simulink model "SF015A_WhlImbRejctn"  (R2013b)
settings: Solver=FixedStepDiscrete  SolverMode=SingleTasking  StartTime=0.0  StopTime=1  FixedStep=0.002  RelTol=1e-3
values from neighbouring files (symbols this model uses):
  ACTIVBANDMAX_ULS_U32 = DataDict.Constant    [SF015A_WhlImbRejctn_DataDict.m]
  ADAPVFILMAX_ULS_F32 = DataDict.Constant    [SF015A_WhlImbRejctn_DataDict.m]
  ARCHGLBPRM_180OVERPI_ULS_F32 = DataDict.Constant    [SF015A_WhlImbRejctn_DataDict.m]
  ARCHGLBPRM_2MILLISEC_SEC_F32 = DataDict.Constant    [SF015A_WhlImbRejctn_DataDict.m]
  ARCHGLBPRM_2PI_ULS_F32 = DataDict.Constant    [SF015A_WhlImbRejctn_DataDict.m]
  ARCHGLBPRM_FLOATZEROTHD_ULS_F32 = DataDict.Constant    [SF015A_WhlImbRejctn_DataDict.m]
  ARCHGLBPRM_PI_ULS_F32 = DataDict.Constant    [SF015A_WhlImbRejctn_DataDict.m]
  ARCHGLBPRM_PIOVER180_ULS_F32 = DataDict.Constant    [SF015A_WhlImbRejctn_DataDict.m]
  ARCHGLBPRM_PIOVER2_ULS_F32 = DataDict.Constant    [SF015A_WhlImbRejctn_DataDict.m]
  CALMINSPERCOUNT_ULS_F32 = DataDict.Constant    [SF015A_WhlImbRejctn_DataDict.m]
  DURATIONDISABLE_CNT_U16 = DataDict.Constant    [SF015A_WhlImbRejctn_DataDict.m]
  FILTWHLSPDMAX_MOTRADPERSEC_F32 = DataDict.Constant    [SF015A_WhlImbRejctn_DataDict.m]
  MICROSECTOMILLISEC_ULS_F32 = DataDict.Constant    [SF015A_WhlImbRejctn_DataDict.m]
  MINSTOMILLISEC_ULS_F32 = DataDict.Constant    [SF015A_WhlImbRejctn_DataDict.m]
  NINETY_ULS_F32 = DataDict.Constant    [SF015A_WhlImbRejctn_DataDict.m]
  NODEBSTEP_CNT_U16 = DataDict.Constant    [SF015A_WhlImbRejctn_DataDict.m]
  NROFDLY_CNT_U08 = DataDict.Constant    [SF015A_WhlImbRejctn_DataDict.m]
  ONEHALF_ULS_F32 = DataDict.Constant    [SF015A_WhlImbRejctn_DataDict.m]
  ONEHUNDRED_ULS_F32 = DataDict.Constant    [SF015A_WhlImbRejctn_DataDict.m]
  ONEOVRTHREE_ULS_F32 = DataDict.Constant    [SF015A_WhlImbRejctn_DataDict.m]
  ONEOVRTWENTY_ULS_F32 = DataDict.Constant    [SF015A_WhlImbRejctn_DataDict.m]
  ONETHOUSAND_ULS_F32 = DataDict.Constant    [SF015A_WhlImbRejctn_DataDict.m]
  PEAKMAX_ULS_F32 = DataDict.Constant    [SF015A_WhlImbRejctn_DataDict.m]
  PEAKMIN_ULS_F32 = DataDict.Constant    [SF015A_WhlImbRejctn_DataDict.m]
  PHAADJMAX_ULS_F32 = DataDict.Constant    [SF015A_WhlImbRejctn_DataDict.m]
  PITIMESSAMPLETIME_ULS_F32 = DataDict.Constant    [SF015A_WhlImbRejctn_DataDict.m]
  STOREDMINSPERCOUNT_ULS_F32 = DataDict.Constant    [SF015A_WhlImbRejctn_DataDict.m]
  TWO_ULS_F32 = DataDict.Constant    [SF015A_WhlImbRejctn_DataDict.m]
  TWOOVRTHREE_ULS_F32 = DataDict.Constant    [SF015A_WhlImbRejctn_DataDict.m]
  WhlImbRejctnAdpvFac = DataDict.Calibration    [SF015A_WhlImbRejctn_DataDict.m]
  WhlImbRejctnAutScaEna = DataDict.Calibration    [SF015A_WhlImbRejctn_DataDict.m]
  WhlImbRejctnAutScaTar = DataDict.Calibration    [SF015A_WhlImbRejctn_DataDict.m]
  WhlImbRejctnCurrMgnSlewPerLoop = DataDict.Calibration    [SF015A_WhlImbRejctn_DataDict.m]
  WhlImbRejctnDcTrendFltRcvryDly = DataDict.Calibration    [SF015A_WhlImbRejctn_DataDict.m]
  WhlImbRejctnDcTrendFltRcvryNegStep = DataDict.Calibration    [SF015A_WhlImbRejctn_DataDict.m]
  WhlImbRejctnDcTrendFltRcvryPosStep = DataDict.Calibration    [SF015A_WhlImbRejctn_DataDict.m]
  WhlImbRejctnDcTrendFltRcvryThd = DataDict.Calibration    [SF015A_WhlImbRejctn_DataDict.m]
  WhlImbRejctnDcTrendTh2Tq = DataDict.Calibration    [SF015A_WhlImbRejctn_DataDict.m]
  WhlImbRejctnDcTrendThTq = DataDict.Calibration    [SF015A_WhlImbRejctn_DataDict.m]
  WhlImbRejctnDcTrendTi2Sec = DataDict.Calibration    [SF015A_WhlImbRejctn_DataDict.m]
  WhlImbRejctnDcTrendTiSec = DataDict.Calibration    [SF015A_WhlImbRejctn_DataDict.m]
  WhlImbRejctnEnaSlewPerLoop = DataDict.Calibration    [SF015A_WhlImbRejctn_DataDict.m]
  WhlImbRejctnFctEna = DataDict.Calibration    [SF015A_WhlImbRejctn_DataDict.m]
  WhlImbRejctnFrqDiagcAmpThd = DataDict.Calibration    [SF015A_WhlImbRejctn_DataDict.m]
  WhlImbRejctnFrqDiagcEna = DataDict.Calibration    [SF015A_WhlImbRejctn_DataDict.m]
  WhlImbRejctnFrqDiagcFltRcvryDly = DataDict.Calibration    [SF015A_WhlImbRejctn_DataDict.m]
  WhlImbRejctnFrqDiagcFltRcvryNegStep = DataDict.Calibration    [SF015A_WhlImbRejctn_DataDict.m]
  WhlImbRejctnFrqDiagcFltRcvryPosStep = DataDict.Calibration    [SF015A_WhlImbRejctn_DataDict.m]
  WhlImbRejctnFrqDiagcFltRcvryThd = DataDict.Calibration    [SF015A_WhlImbRejctn_DataDict.m]
  WhlImbRejctnFrqDiagcThd = DataDict.Calibration    [SF015A_WhlImbRejctn_DataDict.m]
  WhlImbRejctnFrqDiagcTout = DataDict.Calibration    [SF015A_WhlImbRejctn_DataDict.m]
  WhlImbRejctnFrqDiagcUgrPoleMgn = DataDict.Calibration    [SF015A_WhlImbRejctn_DataDict.m]
  WhlImbRejctnFrqScaTblX = DataDict.Calibration    [SF015A_WhlImbRejctn_DataDict.m]
  WhlImbRejctnMaxDurn = DataDict.Calibration    [SF015A_WhlImbRejctn_DataDict.m]
  WhlImbRejctnMaxMgn = DataDict.Calibration    [SF015A_WhlImbRejctn_DataDict.m]
  WhlImbRejctnMaxMgnFltNegStep = DataDict.Calibration    [SF015A_WhlImbRejctn_DataDict.m]
  WhlImbRejctnMaxMgnFltPosStep = DataDict.Calibration    [SF015A_WhlImbRejctn_DataDict.m]
  WhlImbRejctnMaxMgnFltRcvryDly = DataDict.Calibration    [SF015A_WhlImbRejctn_DataDict.m]
  WhlImbRejctnMaxMgnFltRcvryNegStep = DataDict.Calibration    [SF015A_WhlImbRejctn_DataDict.m]
  WhlImbRejctnMaxMgnFltRcvryPosStep = DataDict.Calibration    [SF015A_WhlImbRejctn_DataDict.m]
  WhlImbRejctnMaxMgnFltRcvryThd = DataDict.Calibration    [SF015A_WhlImbRejctn_DataDict.m]
  WhlImbRejctnMaxMgnFltThd = DataDict.Calibration    [SF015A_WhlImbRejctn_DataDict.m]
  WhlImbRejctnMgnEstimnDeltaSca = DataDict.Calibration    [SF015A_WhlImbRejctn_DataDict.m]
  WhlImbRejctnMgnEstimnDiThd = DataDict.Calibration    [SF015A_WhlImbRejctn_DataDict.m]
  WhlImbRejctnMgnEstimnEnaThd = DataDict.Calibration    [SF015A_WhlImbRejctn_DataDict.m]
  WhlImbRejctnMgnEstimnFrq = DataDict.Calibration    [SF015A_WhlImbRejctn_DataDict.m]
  WhlImbRejctnMgnEstimnFrqDelta = DataDict.Calibration    [SF015A_WhlImbRejctn_DataDict.m]
  WhlImbRejctnMgnEstimnLeak = DataDict.Calibration    [SF015A_WhlImbRejctn_DataDict.m]
  WhlImbRejctnRampDwnTi = DataDict.Calibration    [SF015A_WhlImbRejctn_DataDict.m]
  WhlImbRejctnScaCncl = DataDict.Calibration    [SF015A_WhlImbRejctn_DataDict.m]
  WhlImbRejctnUgrPoleMgn = DataDict.Calibration    [SF015A_WhlImbRejctn_DataDict.m]
  WhlImbRejctnVehSpdEna = DataDict.Calibration    [SF015A_WhlImbRejctn_DataDict.m]
  WhlImbRejctnWhlSpdCorrlnFltRcvryDly = DataDict.Calibration    [SF015A_WhlImbRejctn_DataDict.m]
  WhlImbRejctnWhlSpdCorrlnFltRcvryNegStep = DataDict.Calibration    [SF015A_WhlImbRejctn_DataDict.m]
  WhlImbRejctnWhlSpdCorrlnFltRcvryPosStep = DataDict.Calibration    [SF015A_WhlImbRejctn_DataDict.m]
  WhlImbRejctnWhlSpdCorrlnFltRcvryThd = DataDict.Calibration    [SF015A_WhlImbRejctn_DataDict.m]
  WhlImbRejctnWhlSpdCorrlnThd = DataDict.Calibration    [SF015A_WhlImbRejctn_DataDict.m]
  WhlImbRejctnWhlSpdCorrlnTi = DataDict.Calibration    [SF015A_WhlImbRejctn_DataDict.m]
  WIRCMDMAX_MOTNWTMTR_F32 = DataDict.Constant    [SF015A_WhlImbRejctn_DataDict.m]
  ZERO_ULS_F32 = DataDict.Constant    [SF015A_WhlImbRejctn_DataDict.m]
undefined symbols (not defined in the file or in its folder): Cntr, NtcNr1, NvmGetErrSts1, SigQlfr1, Sts, SysSt1
libraries: simulink x32, FixdToFloat x32, Fil x20, NxtrLim x15, NxtrNvM x12, NxtrAbslt x8, NxtrMath x7, NxtrMax x6, NxtrMin x4, FloatToFixd x2, LnrIntrpn x2, NxtrSign x1
(part 2 of 12)

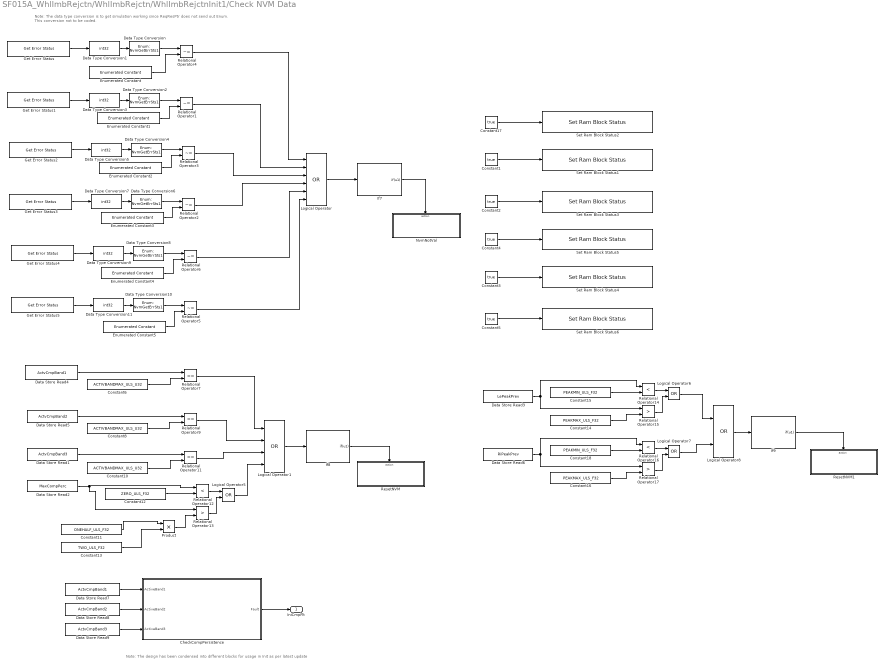
== system SF015A_WhlImbRejctn/WhlImbRejctn/WhlImbRejctnInit1/Check NVM Data ==
  note: Note: The data type conversion is to get simulation working since ReqResPtr does not send out Enum. This
      | conversion not to be coded.
  note: Note: The design has been condensed into different blocks for usage in Init as per latest update
  CheckCompPersistence : Subsystem
  Constant{1..5,17} (6 alike) : Constant  Value=true  OutDataTypeStr=boolean
      settings: AttributesFormatString=%<OutDataTypeStr>
  Constant10 : Constant  RequirementInfo="{'linktype_rmi_doors' '0000ba59 (/E-STEER Core/SubSystem Specifications/Application Functions/SF011A Learned EOT Limits)' '#SF011A_70' 'true' 'REQ:  SF011A_70' '' ; 'linktype_rmi_doors' '0000ba59 (/E-STEER Core/SubSystem Specifications/Application Functions/SF011A Learned EOT Limits)' '#SF011A_71' 'true' 'REQ:  SF011A_71' '' ; 'linktype_rmi_doors' '0000ba59 (/E-STEER Core/SubSystem Specifications/Application Functions/SF011A Learned EOT Limits)' '#SF011A_49' 'true' 'REQ:  SF011A_49' '' } %GIDa_dac22d33_84e0_4d43_9baa_6580695156ec"  Value=ACTIVBANDMAX_ULS_U32
  Constant11 : Constant  RequirementInfo="{'linktype_rmi_doors' '0000ba59 (/E-STEER Core/SubSystem Specifications/Application Functions/SF011A Learned EOT Limits)' '#SF011A_70' 'true' 'REQ:  SF011A_70' '' ; 'linktype_rmi_doors' '0000ba59 (/E-STEER Core/SubSystem Specifications/Application Functions/SF011A Learned EOT Limits)' '#SF011A_71' 'true' 'REQ:  SF011A_71' '' ; 'linktype_rmi_doors' '0000ba59 (/E-STEER Core/SubSystem Specifications/Application Functions/SF011A Learned EOT Limits)' '#SF011A_49' 'true' 'REQ:  SF011A_49' '' } %GIDa_b70b5de3_e4e7_4656_8a10_81d881ba1c41"  Value=ONEHALF_ULS_F32
  Constant12 : Constant  RequirementInfo="{'linktype_rmi_doors' '0000ba59 (/E-STEER Core/SubSystem Specifications/Application Functions/SF011A Learned EOT Limits)' '#SF011A_70' 'true' 'REQ:  SF011A_70' '' ; 'linktype_rmi_doors' '0000ba59 (/E-STEER Core/SubSystem Specifications/Application Functions/SF011A Learned EOT Limits)' '#SF011A_71' 'true' 'REQ:  SF011A_71' '' ; 'linktype_rmi_doors' '0000ba59 (/E-STEER Core/SubSystem Specifications/Application Functions/SF011A Learned EOT Limits)' '#SF011A_48' 'true' 'REQ:  SF011A_48' '' } %GIDa_d9980660_ddd4_4231_a48f_0f3c433b1d8f"  Value=ZERO_ULS_F32
  Constant13 : Constant  RequirementInfo="{'linktype_rmi_doors' '0000ba59 (/E-STEER Core/SubSystem Specifications/Application Functions/SF011A Learned EOT Limits)' '#SF011A_70' 'true' 'REQ:  SF011A_70' '' ; 'linktype_rmi_doors' '0000ba59 (/E-STEER Core/SubSystem Specifications/Application Functions/SF011A Learned EOT Limits)' '#SF011A_71' 'true' 'REQ:  SF011A_71' '' ; 'linktype_rmi_doors' '0000ba59 (/E-STEER Core/SubSystem Specifications/Application Functions/SF011A Learned EOT Limits)' '#SF011A_49' 'true' 'REQ:  SF011A_49' '' } %GIDa_8a202516_8579_4314_b780_b551ef6a9ea7"  Value=TWO_ULS_F32
  Constant14 : Constant  RequirementInfo="{'linktype_rmi_doors' '0000ba59 (/E-STEER Core/SubSystem Specifications/Application Functions/SF011A Learned EOT Limits)' '#SF011A_70' 'true' 'REQ:  SF011A_70' '' ; 'linktype_rmi_doors' '0000ba59 (/E-STEER Core/SubSystem Specifications/Application Functions/SF011A Learned EOT Limits)' '#SF011A_71' 'true' 'REQ:  SF011A_71' '' ; 'linktype_rmi_doors' '0000ba59 (/E-STEER Core/SubSystem Specifications/Application Functions/SF011A Learned EOT Limits)' '#SF011A_49' 'true' 'REQ:  SF011A_49' '' } %GIDa_73aa9993_742b_457a_81a0_f953eb76670e"  Value=PEAKMAX_ULS_F32
  Constant15 : Constant  RequirementInfo="{'linktype_rmi_doors' '0000ba59 (/E-STEER Core/SubSystem Specifications/Application Functions/SF011A Learned EOT Limits)' '#SF011A_70' 'true' 'REQ:  SF011A_70' '' ; 'linktype_rmi_doors' '0000ba59 (/E-STEER Core/SubSystem Specifications/Application Functions/SF011A Learned EOT Limits)' '#SF011A_71' 'true' 'REQ:  SF011A_71' '' ; 'linktype_rmi_doors' '0000ba59 (/E-STEER Core/SubSystem Specifications/Application Functions/SF011A Learned EOT Limits)' '#SF011A_48' 'true' 'REQ:  SF011A_48' '' } %GIDa_1412b3b4_8a5a_4483_b46c_39b8aea63137"  Value=PEAKMIN_ULS_F32
  Constant16 : Constant  RequirementInfo="{'linktype_rmi_doors' '0000ba59 (/E-STEER Core/SubSystem Specifications/Application Functions/SF011A Learned EOT Limits)' '#SF011A_70' 'true' 'REQ:  SF011A_70' '' ; 'linktype_rmi_doors' '0000ba59 (/E-STEER Core/SubSystem Specifications/Application Functions/SF011A Learned EOT Limits)' '#SF011A_71' 'true' 'REQ:  SF011A_71' '' ; 'linktype_rmi_doors' '0000ba59 (/E-STEER Core/SubSystem Specifications/Application Functions/SF011A Learned EOT Limits)' '#SF011A_49' 'true' 'REQ:  SF011A_49' '' } %GIDa_fb2105b3_9180_4cca_ab02_2c62039e61f3"  Value=PEAKMAX_ULS_F32
  Constant18 : Constant  RequirementInfo="{'linktype_rmi_doors' '0000ba59 (/E-STEER Core/SubSystem Specifications/Application Functions/SF011A Learned EOT Limits)' '#SF011A_70' 'true' 'REQ:  SF011A_70' '' ; 'linktype_rmi_doors' '0000ba59 (/E-STEER Core/SubSystem Specifications/Application Functions/SF011A Learned EOT Limits)' '#SF011A_71' 'true' 'REQ:  SF011A_71' '' ; 'linktype_rmi_doors' '0000ba59 (/E-STEER Core/SubSystem Specifications/Application Functions/SF011A Learned EOT Limits)' '#SF011A_48' 'true' 'REQ:  SF011A_48' '' } %GIDa_e66c83e2_3c4a_4c53_aaa1_18a5c79d3e74"  Value=PEAKMIN_ULS_F32
  Constant6 : Constant  RequirementInfo="{'linktype_rmi_doors' '0000ba59 (/E-STEER Core/SubSystem Specifications/Application Functions/SF011A Learned EOT Limits)' '#SF011A_70' 'true' 'REQ:  SF011A_70' '' ; 'linktype_rmi_doors' '0000ba59 (/E-STEER Core/SubSystem Specifications/Application Functions/SF011A Learned EOT Limits)' '#SF011A_71' 'true' 'REQ:  SF011A_71' '' ; 'linktype_rmi_doors' '0000ba59 (/E-STEER Core/SubSystem Specifications/Application Functions/SF011A Learned EOT Limits)' '#SF011A_49' 'true' 'REQ:  SF011A_49' '' } %GIDa_8360f5ba_58c9_48ae_bbc1_d6eb240405df"  Value=ACTIVBANDMAX_ULS_U32
  Constant8 : Constant  RequirementInfo="{'linktype_rmi_doors' '0000ba59 (/E-STEER Core/SubSystem Specifications/Application Functions/SF011A Learned EOT Limits)' '#SF011A_70' 'true' 'REQ:  SF011A_70' '' ; 'linktype_rmi_doors' '0000ba59 (/E-STEER Core/SubSystem Specifications/Application Functions/SF011A Learned EOT Limits)' '#SF011A_71' 'true' 'REQ:  SF011A_71' '' ; 'linktype_rmi_doors' '0000ba59 (/E-STEER Core/SubSystem Specifications/Application Functions/SF011A Learned EOT Limits)' '#SF011A_49' 'true' 'REQ:  SF011A_49' '' } %GIDa_5c7deeb0_1ebc_45b4_93cb_ec8df33bc324"  Value=ACTIVBANDMAX_ULS_U32
  Data Store Read1 : DataStoreRead  RequirementInfo="{'linktype_rmi_doors' '0000ba59 (/E-STEER Core/SubSystem Specifications/Application Functions/SF011A Learned EOT Limits)' '#SF011A_70' 'true' 'REQ:  SF011A_70' '' ; 'linktype_rmi_doors' '0000ba59 (/E-STEER Core/SubSystem Specifications/Application Functions/SF011A Learned EOT Limits)' '#SF011A_71' 'true' 'REQ:  SF011A_71' '' } %GIDa_ec34064d_8d90_476a_a13b_dfcebb6e1578"  DataStoreName=ActvCmpBand3
  Data Store Read2 : DataStoreRead  RequirementInfo="{'linktype_rmi_doors' '0000ba59 (/E-STEER Core/SubSystem Specifications/Application Functions/SF011A Learned EOT Limits)' '#SF011A_70' 'true' 'REQ:  SF011A_70' '' ; 'linktype_rmi_doors' '0000ba59 (/E-STEER Core/SubSystem Specifications/Application Functions/SF011A Learned EOT Limits)' '#SF011A_71' 'true' 'REQ:  SF011A_71' '' } %GIDa_c9bc2b23_4b2d_4415_bc50_be739cb942b2"  DataStoreName=MaxCompPerc
  Data Store Read3 : DataStoreRead  RequirementInfo="{'linktype_rmi_doors' '0000ba59 (/E-STEER Core/SubSystem Specifications/Application Functions/SF011A Learned EOT Limits)' '#SF011A_70' 'true' 'REQ:  SF011A_70' '' ; 'linktype_rmi_doors' '0000ba59 (/E-STEER Core/SubSystem Specifications/Application Functions/SF011A Learned EOT Limits)' '#SF011A_71' 'true' 'REQ:  SF011A_71' '' } %GIDa_b09638af_4375_4cc5_b3f9_eff43fa8b240"  DataStoreName=LePeakPrev
  Data Store Read4 : DataStoreRead  RequirementInfo="{'linktype_rmi_doors' '0000ba59 (/E-STEER Core/SubSystem Specifications/Application Functions/SF011A Learned EOT Limits)' '#SF011A_70' 'true' 'REQ:  SF011A_70' '' ; 'linktype_rmi_doors' '0000ba59 (/E-STEER Core/SubSystem Specifications/Application Functions/SF011A Learned EOT Limits)' '#SF011A_71' 'true' 'REQ:  SF011A_71' '' } %GIDa_a896886f_cd25_4b88_9045_5429e28523e8"  DataStoreName=ActvCmpBand1
  Data Store Read5 : DataStoreRead  RequirementInfo="{'linktype_rmi_doors' '0000ba59 (/E-STEER Core/SubSystem Specifications/Application Functions/SF011A Learned EOT Limits)' '#SF011A_70' 'true' 'REQ:  SF011A_70' '' ; 'linktype_rmi_doors' '0000ba59 (/E-STEER Core/SubSystem Specifications/Application Functions/SF011A Learned EOT Limits)' '#SF011A_71' 'true' 'REQ:  SF011A_71' '' } %GIDa_49f944b4_3c4a_4d70_b0f8_71dc9df1d416"  DataStoreName=ActvCmpBand2
  Data Store Read6 : DataStoreRead  RequirementInfo="{'linktype_rmi_doors' '0000ba59 (/E-STEER Core/SubSystem Specifications/Application Functions/SF011A Learned EOT Limits)' '#SF011A_70' 'true' 'REQ:  SF011A_70' '' ; 'linktype_rmi_doors' '0000ba59 (/E-STEER Core/SubSystem Specifications/Application Functions/SF011A Learned EOT Limits)' '#SF011A_71' 'true' 'REQ:  SF011A_71' '' } %GIDa_db267250_3306_4bc6_b10d_eb14da1fa863"  DataStoreName=RiPeakPrev
  Data Store Read7 : DataStoreRead  Priority=3  DataStoreName=ActvCmpBand1
      settings: AttributesFormatString=Priority=%<Priority>
  Data Store Read8 : DataStoreRead  Priority=3  DataStoreName=ActvCmpBand2
      settings: AttributesFormatString=Priority=%<Priority>
  Data Store Read9 : DataStoreRead  Priority=3  DataStoreName=ActvCmpBand3
      settings: AttributesFormatString=Priority=%<Priority>
  Data Type Conversion : DataTypeConversion  RequirementInfo="{'linktype_rmi_doors' '0000ba59 (/E-STEER Core/SubSystem Specifications/Application Functions/SF011A Learned EOT Limits)' '#SF011A_124' 'true' 'REQ:  SF011A_124' '' } %GIDa_40af021a_ef54_4ec7_b6de_237be91b60fa"  OutDataTypeStr=Enum: NvmGetErrSts1
  Data Type Conversion1 : DataTypeConversion  RequirementInfo="{'linktype_rmi_doors' '0000ba59 (/E-STEER Core/SubSystem Specifications/Application Functions/SF011A Learned EOT Limits)' '#SF011A_124' 'true' 'REQ:  SF011A_124' '' } %GIDa_97cfbfab_5bcd_4235_a187_9f25ba5a5ff5"  OutDataTypeStr=int32
  Data Type Conversion10 : DataTypeConversion  RequirementInfo="{'linktype_rmi_doors' '0000ba59 (/E-STEER Core/SubSystem Specifications/Application Functions/SF011A Learned EOT Limits)' '#SF011A_124' 'true' 'REQ:  SF011A_124' '' } %GIDa_d1594883_ae26_4fe8_b2c9_9956f34c5b40"  OutDataTypeStr=Enum: NvmGetErrSts1
  Data Type Conversion11 : DataTypeConversion  RequirementInfo="{'linktype_rmi_doors' '0000ba59 (/E-STEER Core/SubSystem Specifications/Application Functions/SF011A Learned EOT Limits)' '#SF011A_124' 'true' 'REQ:  SF011A_124' '' } %GIDa_86b4411a_f525_417b_8f1b_33407c25bf86"  OutDataTypeStr=int32
  Data Type Conversion2 : DataTypeConversion  RequirementInfo="{'linktype_rmi_doors' '0000ba59 (/E-STEER Core/SubSystem Specifications/Application Functions/SF011A Learned EOT Limits)' '#SF011A_124' 'true' 'REQ:  SF011A_124' '' } %GIDa_71155e7c_4e44_40ff_94f4_b9d7723c530e"  OutDataTypeStr=Enum: NvmGetErrSts1
  Data Type Conversion3 : DataTypeConversion  RequirementInfo="{'linktype_rmi_doors' '0000ba59 (/E-STEER Core/SubSystem Specifications/Application Functions/SF011A Learned EOT Limits)' '#SF011A_124' 'true' 'REQ:  SF011A_124' '' } %GIDa_b9c1508a_f5ac_4de0_ab2d_9795f69e770d"  OutDataTypeStr=int32
  Data Type Conversion4 : DataTypeConversion  RequirementInfo="{'linktype_rmi_doors' '0000ba59 (/E-STEER Core/SubSystem Specifications/Application Functions/SF011A Learned EOT Limits)' '#SF011A_124' 'true' 'REQ:  SF011A_124' '' } %GIDa_abad9cc4_b739_49e2_b051_31edac34df3e"  OutDataTypeStr=Enum: NvmGetErrSts1
  Data Type Conversion5 : DataTypeConversion  RequirementInfo="{'linktype_rmi_doors' '0000ba59 (/E-STEER Core/SubSystem Specifications/Application Functions/SF011A Learned EOT Limits)' '#SF011A_124' 'true' 'REQ:  SF011A_124' '' } %GIDa_63d91e5a_8420_42e2_a9f3_80e22cdf1e1c"  OutDataTypeStr=int32
  Data Type Conversion6 : DataTypeConversion  RequirementInfo="{'linktype_rmi_doors' '0000ba59 (/E-STEER Core/SubSystem Specifications/Application Functions/SF011A Learned EOT Limits)' '#SF011A_124' 'true' 'REQ:  SF011A_124' '' } %GIDa_6d191fbc_fa3c_4609_af11_f3505129a929"  OutDataTypeStr=Enum: NvmGetErrSts1
  Data Type Conversion7 : DataTypeConversion  RequirementInfo="{'linktype_rmi_doors' '0000ba59 (/E-STEER Core/SubSystem Specifications/Application Functions/SF011A Learned EOT Limits)' '#SF011A_124' 'true' 'REQ:  SF011A_124' '' } %GIDa_257ee758_1562_45cc_b25c_78b92d5b7d32"  OutDataTypeStr=int32
  Data Type Conversion8 : DataTypeConversion  RequirementInfo="{'linktype_rmi_doors' '0000ba59 (/E-STEER Core/SubSystem Specifications/Application Functions/SF011A Learned EOT Limits)' '#SF011A_124' 'true' 'REQ:  SF011A_124' '' } %GIDa_a7c9a5b3_e719_4c4f_b06f_c23b0932ba59"  OutDataTypeStr=Enum: NvmGetErrSts1
  Data Type Conversion9 : DataTypeConversion  RequirementInfo="{'linktype_rmi_doors' '0000ba59 (/E-STEER Core/SubSystem Specifications/Application Functions/SF011A Learned EOT Limits)' '#SF011A_124' 'true' 'REQ:  SF011A_124' '' } %GIDa_0f1e9d57_eff5_4620_a47c_e9abcc1d02d7"  OutDataTypeStr=int32
  Enumerated Constant : simulink/Sources/Enumerated Constant  RequirementInfo="{'linktype_rmi_doors' '0000ba59 (/E-STEER Core/SubSystem Specifications/Application Functions/SF011A Learned EOT Limits)' '#SF011A_124' 'true' 'REQ:  SF011A_124' '' } %GIDa_d56addf7_f0d4_4bf6_af4c_9a6eaaf5d064"  OutDataTypeStr=Enum: NvmGetErrSts1  Value=NvmGetErrSts1.REQUEST_OK  SampleTime=inf
  Enumerated Constant1 : simulink/Sources/Enumerated Constant  RequirementInfo="{'linktype_rmi_doors' '0000ba59 (/E-STEER Core/SubSystem Specifications/Application Functions/SF011A Learned EOT Limits)' '#SF011A_124' 'true' 'REQ:  SF011A_124' '' } %GIDa_5e154709_209f_4b86_818d_2a89bf246dcb"  OutDataTypeStr=Enum: NvmGetErrSts1  Value=NvmGetErrSts1.REQUEST_OK  SampleTime=inf
  Enumerated Constant2 : simulink/Sources/Enumerated Constant  RequirementInfo="{'linktype_rmi_doors' '0000ba59 (/E-STEER Core/SubSystem Specifications/Application Functions/SF011A Learned EOT Limits)' '#SF011A_124' 'true' 'REQ:  SF011A_124' '' } %GIDa_b9f04514_19b2_47ae_b701_837fe354ebc7"  OutDataTypeStr=Enum: NvmGetErrSts1  Value=NvmGetErrSts1.REQUEST_OK  SampleTime=inf
  Enumerated Constant3 : simulink/Sources/Enumerated Constant  RequirementInfo="{'linktype_rmi_doors' '0000ba59 (/E-STEER Core/SubSystem Specifications/Application Functions/SF011A Learned EOT Limits)' '#SF011A_124' 'true' 'REQ:  SF011A_124' '' } %GIDa_006fb6d4_b105_4186_b45b_bb6a02141efd"  OutDataTypeStr=Enum: NvmGetErrSts1  Value=NvmGetErrSts1.REQUEST_OK  SampleTime=inf
  Enumerated Constant4 : simulink/Sources/Enumerated Constant  RequirementInfo="{'linktype_rmi_doors' '0000ba59 (/E-STEER Core/SubSystem Specifications/Application Functions/SF011A Learned EOT Limits)' '#SF011A_124' 'true' 'REQ:  SF011A_124' '' } %GIDa_f995986c_c311_4ae9_af99_76f05a8496d8"  OutDataTypeStr=Enum: NvmGetErrSts1  Value=NvmGetErrSts1.REQUEST_OK  SampleTime=inf
  Enumerated Constant5 : simulink/Sources/Enumerated Constant  RequirementInfo="{'linktype_rmi_doors' '0000ba59 (/E-STEER Core/SubSystem Specifications/Application Functions/SF011A Learned EOT Limits)' '#SF011A_124' 'true' 'REQ:  SF011A_124' '' } %GIDa_f15c7506_b69b_4bb1_898d_0e3ef15f7387"  OutDataTypeStr=Enum: NvmGetErrSts1  Value=NvmGetErrSts1.REQUEST_OK  SampleTime=inf
  Get Error Status : NxtrNvM/Get Error Status  RequirementInfo="{'linktype_rmi_doors' '0000ba59 (/E-STEER Core/SubSystem Specifications/Application Functions/SF011A Learned EOT Limits)' '#SF011A_124' 'true' 'REQ:  SF011A_124' '' } %GIDa_553b790d_fe60_40ec_8b91_d9fbb8c02471"  FuncName=Get Error Status  NvMBlockName=ActvCmpBand1  VoidFuncRtn=on  ReqResPtr_DSN=NvMGES_ReqResPtr1  Return_DSN=NvMGES_Return
      settings: AttributesFormatString=%<FuncName>
  Get Error Status1 : NxtrNvM/Get Error Status  RequirementInfo="{'linktype_rmi_doors' '0000ba59 (/E-STEER Core/SubSystem Specifications/Application Functions/SF011A Learned EOT Limits)' '#SF011A_124' 'true' 'REQ:  SF011A_124' '' } %GIDa_2abd0d7c_8999_4277_934d_b39154cf423f"  FuncName=Get Error Status  NvMBlockName=ActvCmpBand2  VoidFuncRtn=on  ReqResPtr_DSN=NvMGES_ReqResPtr2  Return_DSN=NvMGES_Return
      settings: AttributesFormatString=%<FuncName>
  Get Error Status2 : NxtrNvM/Get Error Status  RequirementInfo="{'linktype_rmi_doors' '0000ba59 (/E-STEER Core/SubSystem Specifications/Application Functions/SF011A Learned EOT Limits)' '#SF011A_124' 'true' 'REQ:  SF011A_124' '' } %GIDa_b704cbe0_0ff9_45ea_89ac_8ddce2b05c13"  FuncName=Get Error Status  NvMBlockName=ActvCmpBand3  VoidFuncRtn=on  ReqResPtr_DSN=NvMGES_ReqResPtr3  Return_DSN=NvMGES_Return
      settings: AttributesFormatString=%<FuncName>
  Get Error Status3 : NxtrNvM/Get Error Status  RequirementInfo="{'linktype_rmi_doors' '0000ba59 (/E-STEER Core/SubSystem Specifications/Application Functions/SF011A Learned EOT Limits)' '#SF011A_124' 'true' 'REQ:  SF011A_124' '' } %GIDa_06d65f98_25d9_49e6_9db6_cd70c37fa23a"  FuncName=Get Error Status  NvMBlockName=LePeakPrev  VoidFuncRtn=on  ReqResPtr_DSN=NvMGES_ReqResPtr4  Return_DSN=NvMGES_Return
      settings: AttributesFormatString=%<FuncName>
  Get Error Status4 : NxtrNvM/Get Error Status  RequirementInfo="{'linktype_rmi_doors' '0000ba59 (/E-STEER Core/SubSystem Specifications/Application Functions/SF011A Learned EOT Limits)' '#SF011A_124' 'true' 'REQ:  SF011A_124' '' } %GIDa_0df4cd3c_6ba5_402f_93b7_8579f841a241"  FuncName=Get Error Status  NvMBlockName=MaxCompPerc  VoidFuncRtn=on  ReqResPtr_DSN=NvMGES_ReqResPtr5  Return_DSN=NvMGES_Return
      settings: AttributesFormatString=%<FuncName>
  Get Error Status5 : NxtrNvM/Get Error Status  RequirementInfo="{'linktype_rmi_doors' '0000ba59 (/E-STEER Core/SubSystem Specifications/Application Functions/SF011A Learned EOT Limits)' '#SF011A_124' 'true' 'REQ:  SF011A_124' '' } %GIDa_76d426a4_53ff_4480_8e93_077011626842"  FuncName=Get Error Status  NvMBlockName=RiPeakPrev  VoidFuncRtn=on  ReqResPtr_DSN=NvMGES_ReqResPtr6  Return_DSN=NvMGES_Return
      settings: AttributesFormatString=%<FuncName>
  If7 : If  RequirementInfo="{'linktype_rmi_doors' '0000ba59 (/E-STEER Core/SubSystem Specifications/Application Functions/SF011A Learned EOT Limits)' '#SF011A_124' 'true' 'REQ:  SF011A_124' '' } %GIDa_907c88cf_d2cc_420d_8539_4883f54d5bfb"  Priority=0  IfExpression=u1  ShowElse=off
  If8 : If  RequirementInfo="{'linktype_rmi_doors' '0000ba59 (/E-STEER Core/SubSystem Specifications/Application Functions/SF011A Learned EOT Limits)' '#SF011A_124' 'true' 'REQ:  SF011A_124' '' } %GIDa_f83260c7_70fe_47e6_bcfd_8d40190318cc"  Priority=0  IfExpression=u1  ShowElse=off
  If9 : If  RequirementInfo="{'linktype_rmi_doors' '0000ba59 (/E-STEER Core/SubSystem Specifications/Application Functions/SF011A Learned EOT Limits)' '#SF011A_124' 'true' 'REQ:  SF011A_124' '' } %GIDa_2d76ece9_77c8_4d3b_9932_2561659afd1c"  Priority=0  IfExpression=u1  ShowElse=off
  Logical Operator : Logic  RequirementInfo="{'linktype_rmi_doors' '0000ba59 (/E-STEER Core/SubSystem Specifications/Application Functions/SF011A Learned EOT Limits)' '#SF011A_70' 'true' 'REQ:  SF011A_70' '' ; 'linktype_rmi_doors' '0000ba59 (/E-STEER Core/SubSystem Specifications/Application Functions/SF011A Learned EOT Limits)' '#SF011A_71' 'true' 'REQ:  SF011A_71' '' } %GIDa_fbe3003e_bdb5_447d_bc60_e1c843a8f900"  Operator=OR  Inputs=6  AllPortsSameDT=off  OutDataTypeStr=boolean
  Logical Operator1 : Logic  RequirementInfo="{'linktype_rmi_doors' '0000ba59 (/E-STEER Core/SubSystem Specifications/Application Functions/SF011A Learned EOT Limits)' '#SF011A_70' 'true' 'REQ:  SF011A_70' '' ; 'linktype_rmi_doors' '0000ba59 (/E-STEER Core/SubSystem Specifications/Application Functions/SF011A Learned EOT Limits)' '#SF011A_71' 'true' 'REQ:  SF011A_71' '' } %GIDa_6b27fa6d_5a8c_4b6e_9ec1_9ce35c4a7e3a"  Operator=OR  Inputs=4  AllPortsSameDT=off  OutDataTypeStr=boolean
  Logical Operator5 : Logic  RequirementInfo="{'linktype_rmi_doors' '0000ba59 (/E-STEER Core/SubSystem Specifications/Application Functions/SF011A Learned EOT Limits)' '#SF011A_70' 'true' 'REQ:  SF011A_70' '' ; 'linktype_rmi_doors' '0000ba59 (/E-STEER Core/SubSystem Specifications/Application Functions/SF011A Learned EOT Limits)' '#SF011A_71' 'true' 'REQ:  SF011A_71' '' } %GIDa_ff21cde4_e337_434b_869a_bfcb48407868"  Operator=OR  AllPortsSameDT=off  OutDataTypeStr=boolean
  Logical Operator6 : Logic  RequirementInfo="{'linktype_rmi_doors' '0000ba59 (/E-STEER Core/SubSystem Specifications/Application Functions/SF011A Learned EOT Limits)' '#SF011A_70' 'true' 'REQ:  SF011A_70' '' ; 'linktype_rmi_doors' '0000ba59 (/E-STEER Core/SubSystem Specifications/Application Functions/SF011A Learned EOT Limits)' '#SF011A_71' 'true' 'REQ:  SF011A_71' '' } %GIDa_22490e7d_9c19_4dde_99cc_08f0ef37cc37"  Operator=OR  AllPortsSameDT=off  OutDataTypeStr=boolean
  Logical Operator7 : Logic  RequirementInfo="{'linktype_rmi_doors' '0000ba59 (/E-STEER Core/SubSystem Specifications/Application Functions/SF011A Learned EOT Limits)' '#SF011A_70' 'true' 'REQ:  SF011A_70' '' ; 'linktype_rmi_doors' '0000ba59 (/E-STEER Core/SubSystem Specifications/Application Functions/SF011A Learned EOT Limits)' '#SF011A_71' 'true' 'REQ:  SF011A_71' '' } %GIDa_0952c7bd_6ac0_4128_a8d2_c4d9c59f71ec"  Operator=OR  AllPortsSameDT=off  OutDataTypeStr=boolean
  Logical Operator8 : Logic  RequirementInfo="{'linktype_rmi_doors' '0000ba59 (/E-STEER Core/SubSystem Specifications/Application Functions/SF011A Learned EOT Limits)' '#SF011A_70' 'true' 'REQ:  SF011A_70' '' ; 'linktype_rmi_doors' '0000ba59 (/E-STEER Core/SubSystem Specifications/Application Functions/SF011A Learned EOT Limits)' '#SF011A_71' 'true' 'REQ:  SF011A_71' '' } %GIDa_f87f89e5_1919_41e6_b4c5_1617d795e711"  Operator=OR  AllPortsSameDT=off  OutDataTypeStr=boolean
  NvmNotVal : Subsystem  RequirementInfo="{'linktype_rmi_doors' '0000ba59 (/E-STEER Core/SubSystem Specifications/Application Functions/SF011A Learned EOT Limits)' '#SF011A_124' 'true' 'REQ:  SF011A_124' '' } %GIDa_f6393af9_0f72_404f_ae39_57d92493339f"  TreatAsAtomicUnit=on
  Product : Product
  Relational Operator1 : RelationalOperator  RequirementInfo="{'linktype_rmi_doors' '0000ba59 (/E-STEER Core/SubSystem Specifications/Application Functions/SF011A Learned EOT Limits)' '#SF011A_124' 'true' 'REQ:  SF011A_124' '' } %GIDa_7a10770e_4cc4_43da_8b61_7817b3645f3e"  Operator=~=  OutDataTypeStr=boolean
  Relational Operator11 : RelationalOperator  RequirementInfo="{'linktype_rmi_doors' '0000ba59 (/E-STEER Core/SubSystem Specifications/Application Functions/SF011A Learned EOT Limits)' '#SF011A_70' 'true' 'REQ:  SF011A_70' '' ; 'linktype_rmi_doors' '0000ba59 (/E-STEER Core/SubSystem Specifications/Application Functions/SF011A Learned EOT Limits)' '#SF011A_71' 'true' 'REQ:  SF011A_71' '' } %GIDa_9bbcc360_5740_4f1b_a35a_ba783374856a"  Operator===  OutDataTypeStr=boolean
  Relational Operator12 : RelationalOperator  RequirementInfo="{'linktype_rmi_doors' '0000ba59 (/E-STEER Core/SubSystem Specifications/Application Functions/SF011A Learned EOT Limits)' '#SF011A_70' 'true' 'REQ:  SF011A_70' '' ; 'linktype_rmi_doors' '0000ba59 (/E-STEER Core/SubSystem Specifications/Application Functions/SF011A Learned EOT Limits)' '#SF011A_71' 'true' 'REQ:  SF011A_71' '' } %GIDa_a76e833d_5218_4e43_8d52_6f49a79e2f35"  Operator=<  OutDataTypeStr=boolean
  Relational Operator13 : RelationalOperator  RequirementInfo="{'linktype_rmi_doors' '0000ba59 (/E-STEER Core/SubSystem Specifications/Application Functions/SF011A Learned EOT Limits)' '#SF011A_70' 'true' 'REQ:  SF011A_70' '' ; 'linktype_rmi_doors' '0000ba59 (/E-STEER Core/SubSystem Specifications/Application Functions/SF011A Learned EOT Limits)' '#SF011A_71' 'true' 'REQ:  SF011A_71' '' } %GIDa_4a8bae17_bbe3_48ac_9e0a_4fe9b537a9c6"  Operator=>  OutDataTypeStr=boolean
  Relational Operator14 : RelationalOperator  RequirementInfo="{'linktype_rmi_doors' '0000ba59 (/E-STEER Core/SubSystem Specifications/Application Functions/SF011A Learned EOT Limits)' '#SF011A_70' 'true' 'REQ:  SF011A_70' '' ; 'linktype_rmi_doors' '0000ba59 (/E-STEER Core/SubSystem Specifications/Application Functions/SF011A Learned EOT Limits)' '#SF011A_71' 'true' 'REQ:  SF011A_71' '' } %GIDa_654c4bba_0100_4331_8452_58d1590c8b97"  Operator=<  OutDataTypeStr=boolean
  Relational Operator15 : RelationalOperator  RequirementInfo="{'linktype_rmi_doors' '0000ba59 (/E-STEER Core/SubSystem Specifications/Application Functions/SF011A Learned EOT Limits)' '#SF011A_70' 'true' 'REQ:  SF011A_70' '' ; 'linktype_rmi_doors' '0000ba59 (/E-STEER Core/SubSystem Specifications/Application Functions/SF011A Learned EOT Limits)' '#SF011A_71' 'true' 'REQ:  SF011A_71' '' } %GIDa_e495d182_ff98_497d_82f4_fbf92eddef9e"  Operator=>  OutDataTypeStr=boolean
  Relational Operator16 : RelationalOperator  RequirementInfo="{'linktype_rmi_doors' '0000ba59 (/E-STEER Core/SubSystem Specifications/Application Functions/SF011A Learned EOT Limits)' '#SF011A_70' 'true' 'REQ:  SF011A_70' '' ; 'linktype_rmi_doors' '0000ba59 (/E-STEER Core/SubSystem Specifications/Application Functions/SF011A Learned EOT Limits)' '#SF011A_71' 'true' 'REQ:  SF011A_71' '' } %GIDa_956274a6_c5b5_492b_bac4_f5c4aafd6507"  Operator=<  OutDataTypeStr=boolean
  Relational Operator17 : RelationalOperator  RequirementInfo="{'linktype_rmi_doors' '0000ba59 (/E-STEER Core/SubSystem Specifications/Application Functions/SF011A Learned EOT Limits)' '#SF011A_70' 'true' 'REQ:  SF011A_70' '' ; 'linktype_rmi_doors' '0000ba59 (/E-STEER Core/SubSystem Specifications/Application Functions/SF011A Learned EOT Limits)' '#SF011A_71' 'true' 'REQ:  SF011A_71' '' } %GIDa_3a72db96_6452_4e24_94d0_249eb710d610"  Operator=>  OutDataTypeStr=boolean
  Relational Operator2 : RelationalOperator  RequirementInfo="{'linktype_rmi_doors' '0000ba59 (/E-STEER Core/SubSystem Specifications/Application Functions/SF011A Learned EOT Limits)' '#SF011A_124' 'true' 'REQ:  SF011A_124' '' } %GIDa_5de2de92_e34b_43fe_96ff_f0865a87ab82"  Operator=~=  OutDataTypeStr=boolean
  Relational Operator3 : RelationalOperator  RequirementInfo="{'linktype_rmi_doors' '0000ba59 (/E-STEER Core/SubSystem Specifications/Application Functions/SF011A Learned EOT Limits)' '#SF011A_124' 'true' 'REQ:  SF011A_124' '' } %GIDa_26228c4f_e434_4be0_89f8_80cc184ea71e"  Operator=~=  OutDataTypeStr=boolean
  Relational Operator4 : RelationalOperator  RequirementInfo="{'linktype_rmi_doors' '0000ba59 (/E-STEER Core/SubSystem Specifications/Application Functions/SF011A Learned EOT Limits)' '#SF011A_124' 'true' 'REQ:  SF011A_124' '' } %GIDa_240ffe86_9b38_40e3_a7e4_d3f8c5427260"  Operator=~=  OutDataTypeStr=boolean
  Relational Operator5 : RelationalOperator  RequirementInfo="{'linktype_rmi_doors' '0000ba59 (/E-STEER Core/SubSystem Specifications/Application Functions/SF011A Learned EOT Limits)' '#SF011A_124' 'true' 'REQ:  SF011A_124' '' } %GIDa_b573ea29_a443_4995_b5cb_42c21e85357c"  Operator=~=  OutDataTypeStr=boolean
  Relational Operator6 : RelationalOperator  RequirementInfo="{'linktype_rmi_doors' '0000ba59 (/E-STEER Core/SubSystem Specifications/Application Functions/SF011A Learned EOT Limits)' '#SF011A_124' 'true' 'REQ:  SF011A_124' '' } %GIDa_1e1a5ce8_983a_43e0_b428_4480c44996af"  Operator=~=  OutDataTypeStr=boolean
  Relational Operator7 : RelationalOperator  RequirementInfo="{'linktype_rmi_doors' '0000ba59 (/E-STEER Core/SubSystem Specifications/Application Functions/SF011A Learned EOT Limits)' '#SF011A_70' 'true' 'REQ:  SF011A_70' '' ; 'linktype_rmi_doors' '0000ba59 (/E-STEER Core/SubSystem Specifications/Application Functions/SF011A Learned EOT Limits)' '#SF011A_71' 'true' 'REQ:  SF011A_71' '' } %GIDa_ed9b8f8a_c888_45f6_bfd8_2fd8844e647e"  Operator===  OutDataTypeStr=boolean
  Relational Operator9 : RelationalOperator  RequirementInfo="{'linktype_rmi_doors' '0000ba59 (/E-STEER Core/SubSystem Specifications/Application Functions/SF011A Learned EOT Limits)' '#SF011A_70' 'true' 'REQ:  SF011A_70' '' ; 'linktype_rmi_doors' '0000ba59 (/E-STEER Core/SubSystem Specifications/Application Functions/SF011A Learned EOT Limits)' '#SF011A_71' 'true' 'REQ:  SF011A_71' '' } %GIDa_5b0fe435_eb00_4504_b67e_fcbdb6466ad9"  Operator===  OutDataTypeStr=boolean
  ResetNVM : Subsystem  RequirementInfo="{'linktype_rmi_doors' '0000ba59 (/E-STEER Core/SubSystem Specifications/Application Functions/SF011A Learned EOT Limits)' '#SF011A_124' 'true' 'REQ:  SF011A_124' '' } %GIDa_841a7b4b_65c9_4d3a_ad5a_ef4b7fb654a5"  TreatAsAtomicUnit=on
  ResetNVM1 : Subsystem  RequirementInfo="{'linktype_rmi_doors' '0000ba59 (/E-STEER Core/SubSystem Specifications/Application Functions/SF011A Learned EOT Limits)' '#SF011A_124' 'true' 'REQ:  SF011A_124' '' } %GIDa_21072be2_221d_447f_a6c4_95766f8093de"  TreatAsAtomicUnit=on
  Set Ram Block Status1 : NxtrNvM/Set Ram Block Status  FuncName=Set Ram Block Status  NvMBlockName=ActvCmpBand2  VoidFuncRtn=on  BlockChanged_DSN=NvMSRBS_BlockChanged2  Return_DSN=NvMSRBS_Return
      settings: AttributesFormatString=%<FuncName>
  Set Ram Block Status2 : NxtrNvM/Set Ram Block Status  FuncName=Set Ram Block Status  NvMBlockName=ActvCmpBand1  VoidFuncRtn=on  BlockChanged_DSN=NvMSRBS_BlockChanged1  Return_DSN=NvMSRBS_Return
      settings: AttributesFormatString=%<FuncName>
  Set Ram Block Status3 : NxtrNvM/Set Ram Block Status  FuncName=Set Ram Block Status  NvMBlockName=ActvCmpBand3  VoidFuncRtn=on  BlockChanged_DSN=NvMSRBS_BlockChanged3  Return_DSN=NvMSRBS_Return
      settings: AttributesFormatString=%<FuncName>
  Set Ram Block Status4 : NxtrNvM/Set Ram Block Status  FuncName=Set Ram Block Status  NvMBlockName=MaxCompPerc  VoidFuncRtn=on  BlockChanged_DSN=NvMSRBS_BlockChanged5  Return_DSN=NvMSRBS_Return
      settings: AttributesFormatString=%<FuncName>
  Set Ram Block Status5 : NxtrNvM/Set Ram Block Status  FuncName=Set Ram Block Status  NvMBlockName=LePeakPrev  VoidFuncRtn=on  BlockChanged_DSN=NvMSRBS_BlockChanged4  Return_DSN=NvMSRBS_Return
      settings: AttributesFormatString=%<FuncName>
  Set Ram Block Status6 : NxtrNvM/Set Ram Block Status  FuncName=Set Ram Block Status  NvMBlockName=RiPeakPrev  VoidFuncRtn=on  BlockChanged_DSN=NvMSRBS_BlockChanged6  Return_DSN=NvMSRBS_Return
      settings: AttributesFormatString=%<FuncName>
  IniCmpFlt : Outport
  wires:
  Data Type Conversion/1 -> Relational Operator4/1
  Enumerated Constant/1 -> Relational Operator4/2
  Data Type Conversion1/1 -> Data Type Conversion/1
  Relational Operator1/1 -> Logical Operator/2
  Data Type Conversion2/1 -> Relational Operator1/1
  Get Error Status1/1 -> Data Type Conversion3/1
  Data Type Conversion11/1 -> Data Type Conversion10/1
  Data Type Conversion6/1 -> Relational Operator2/1
  Data Type Conversion3/1 -> Data Type Conversion2/1
  Data Type Conversion8/1 -> Relational Operator6/1
  Data Type Conversion7/1 -> Data Type Conversion6/1
  Data Type Conversion10/1 -> Relational Operator5/1
  Data Type Conversion5/1 -> Data Type Conversion4/1
  Data Type Conversion4/1 -> Relational Operator3/1
  Get Error Status4/1 -> Data Type Conversion9/1
  Get Error Status3/1 -> Data Type Conversion7/1
  Get Error Status2/1 -> Data Type Conversion5/1
  Get Error Status/1 -> Data Type Conversion1/1
  Data Type Conversion9/1 -> Data Type Conversion8/1
  Get Error Status5/1 -> Data Type Conversion11/1
  Constant17/1 -> Set Ram Block Status2/1
  Logical Operator/1 -> If7/1
  Relational Operator4/1 -> Logical Operator/1
  Relational Operator3/1 -> Logical Operator/3
  Relational Operator2/1 -> Logical Operator/4
  Relational Operator6/1 -> Logical Operator/5
  Relational Operator5/1 -> Logical Operator/6
  Constant1/1 -> Set Ram Block Status1/1
  Constant2/1 -> Set Ram Block Status3/1
  Constant4/1 -> Set Ram Block Status5/1
  Constant3/1 -> Set Ram Block Status4/1
  Constant5/1 -> Set Ram Block Status6/1
  Data Store Read4/1 -> Relational Operator7/1
  Constant6/1 -> Relational Operator7/2
  Relational Operator7/1 -> Logical Operator1/1
  Data Store Read5/1 -> Relational Operator9/1
  Constant8/1 -> Relational Operator9/2
  Data Store Read1/1 -> Relational Operator11/1
  Constant10/1 -> Relational Operator11/2
  Logical Operator1/1 -> If8/1
  Data Store Read2/1 -> Relational Operator13/1, Relational Operator12/1
  Constant11/1 -> Product/1
  Constant12/1 -> Relational Operator12/2
  Relational Operator12/1 -> Logical Operator5/1
  Relational Operator13/1 -> Logical Operator5/2
  Logical Operator5/1 -> Logical Operator1/4
  Product/1 -> Relational Operator13/2
  Constant13/1 -> Product/2
  Data Store Read3/1 -> Relational Operator14/1, Relational Operator15/1
  Constant14/1 -> Relational Operator15/2
  Constant15/1 -> Relational Operator14/2
  Relational Operator14/1 -> Logical Operator6/1
  Relational Operator15/1 -> Logical Operator6/2
  Logical Operator6/1 -> Logical Operator8/1
  Data Store Read6/1 -> Relational Operator16/1, Relational Operator17/1
  Constant16/1 -> Relational Operator17/2
  Constant18/1 -> Relational Operator16/2
  Relational Operator16/1 -> Logical Operator7/1
  Relational Operator17/1 -> Logical Operator7/2
  Logical Operator7/1 -> Logical Operator8/2
  Logical Operator8/1 -> If9/1
  Relational Operator9/1 -> Logical Operator1/2
  Relational Operator11/1 -> Logical Operator1/3
  If7/1 -> NvmNotVal/Action
  If8/1 -> ResetNVM/Action
  If9/1 -> ResetNVM1/Action
  Data Store Read7/1 -> CheckCompPersistence/1(ActiveBand1)
  Data Store Read8/1 -> CheckCompPersistence/2(ActiveBand2)
  Data Store Read9/1 -> CheckCompPersistence/3(ActiveBand3)
  CheckCompPersistence/1(Fault) -> IniCmpFlt/1
  Enumerated Constant5/1 -> Relational Operator5/2
  Enumerated Constant4/1 -> Relational Operator6/2
  Enumerated Constant3/1 -> Relational Operator2/2
  Enumerated Constant2/1 -> Relational Operator3/2
  Enumerated Constant1/1 -> Relational Operator1/2

== system SF015A_WhlImbRejctn/WhlImbRejctn/WhlImbRejctnInit1/CopyRight2 ==

== system SF015A_WhlImbRejctn/WhlImbRejctn/WhlImbRejctnPer1/Active Rejection Command  ==
  HwTrq_HwNm : Inport
  Enable : Inport  Port=2
  WhlSpdLFilt_RadpS : Inport  Port=3
  WhlSpdRFilt_RadpS : Inport  Port=4
  FreqEst : Inport  Port=5
  Adaptive Filter - FloatingL : Subsystem
  Adaptive Filter - FloatingR : Subsystem
  Add2 : Sum
  Amplitude Calculation : Subsystem
  Constant : Constant  Value=0  OutDataTypeStr=single
  Constant1 : Constant  Value=WIRCMDMAX_MOTNWTMTR_F32
  Constant2 : Constant  Value=WIRCMDMAX_MOTNWTMTR_F32
  Constant3 : Constant  Value=WhlImbRejctnAdpvFac
  Constant5 : Constant  Value=WhlImbRejctnAdpvFac
  Constant6 : Constant  Value=WhlImbRejctnScaCncl
  CopyRight2 : Subsystem  Description=|  mask(Copyright Information){none=on}
      | Copyright info block.                                               
      |                                                                     
      | Place copyright information at the top of every subsystem in design.
      mask prompts: none "No parameters"
      mask help: Place copyright information at the top of every subsystem in design.
      mask Display:
      | NxtrConf = 'Nexteer Confidential';
      | 
      | sys = bdroot; %handle for the current model ("system")
      | first = get_param(sys,'Created');
      | first = first(end-3:end);  %year is last four digits
      | 
      | last = get_param(sys,'LastModifiedDate');
      | if isempty(last)
      |     last = datestr(now,'yyyy');
      | else
      |     last = last(end-3:end);
      | end
      | 
      | if strcmp(first,last)
      |     fprintf('%s -- Copyright %s Nexteer',NxtrConf,first)
      | else
      |     fprintf('%s -- %s%s- %s Nexteer',NxtrConf,char(169),first,last)
      | end
  Data Store Read : DataStoreRead  Priority=1  DataStoreName=PrevHwTq
      settings: AttributesFormatString=%<Priority>
  Data Store Read1 : DataStoreRead  Priority=1  DataStoreName=PrevHwTq
      settings: AttributesFormatString=%<Priority>
  Data Store Write : DataStoreWrite  Priority=2  DataStoreName=PrevHwTq
      settings: AttributesFormatString=%<Priority>
  Data Store Write1 : DataStoreWrite  DataStoreName=dWhlImbRejctnCnclTqOutp
  LimDyn_f1 : NxtrLim/LimDyn_f32
  LimDyn_f32 : NxtrLim/LimDyn_f32
  Phase Adjust - Floating Point : Subsystem
  Product2 : Product
  Unary Minus : UnaryMinus
  Unary Minus1 : UnaryMinus
  WhlImbRejCmd_MtrNm : Outport
  Amp_WhlImbRejctn : Outport  Port=2
  wires:
  FreqEst/1 -> Phase Adjust - Floating Point/2(Signal Frequency [Hz])
  Constant2/1 -> LimDyn_f32/3, Unary Minus1/1
  Unary Minus1/1 -> LimDyn_f32/2
  Data Store Read/1 -> Adaptive Filter - FloatingL/2(PrevEpsilon)
  Constant3/1 -> Adaptive Filter - FloatingL/3(AdaptiveMu)
  WhlSpdLFilt_RadpS/1 -> Adaptive Filter - FloatingL/4(x Ref)
  Data Store Read1/1 -> Adaptive Filter - FloatingR/2(PrevEpsilon)
  Constant5/1 -> Adaptive Filter - FloatingR/3(AdaptiveMu)
  WhlSpdRFilt_RadpS/1 -> Adaptive Filter - FloatingR/4(x Ref)
  Add2/1 -> Phase Adjust - Floating Point/1(Input Signal)
  Constant6/1 -> Product2/2
  Unary Minus/1 -> Product2/1
  Enable/1 -> [Enable]
  [Enable] -> Adaptive Filter - FloatingL/1(Enable)
  [Enable] -> Adaptive Filter - FloatingR/1(Enable)
  Adaptive Filter - FloatingL/1(output) -> [LeOutput]
  [LeOutput] -> Add2/1
  [RiOutput] -> Add2/2
  Adaptive Filter - FloatingR/1(output) -> [RiOutput]
  Phase Adjust - Floating Point/1(Adjusted Signal) -> Unary Minus/1
  HwTrq_HwNm/1 -> Data Store Write/1
  Product2/1 -> LimDyn_f32/1, Data Store Write1/1
  LimDyn_f32/1 -> WhlImbRejCmd_MtrNm/1, Amplitude Calculation/1(Input)
  LimDyn_f1/1 -> Amp_WhlImbRejctn/1
  Amplitude Calculation/1(Amp) -> LimDyn_f1/1
  Constant/1 -> LimDyn_f1/2
  Constant1/1 -> LimDyn_f1/3

== system SF015A_WhlImbRejctn/WhlImbRejctn/WhlImbRejctnPer1/CopyRight2 ==

== system SF015A_WhlImbRejctn/WhlImbRejctn/WhlImbRejctnPer1/Determine Enabled Amt ==
  FreqEstAvg_Hz1 : Inport
  WhlSpdLFilt : Inport  Port=2
  WhlSpdRFilt : Inport  Port=3
  VehSpd : Inport  Port=4
  VehspdValid : Inport  Port=5
  WhlImbRejctnCustEna : Inport  Port=6
  WhlImbRejctnDi : Inport  Port=7
  System_State : Inport  Port=8
  CurrMgnSlewRate : Inport  Port=9
  EnaSlewRate : Inport  Port=10
  Calculate Enable1 : Subsystem
  CopyRight2 : Subsystem  Description=|  mask(Copyright Information){none=on}
      | Copyright info block.                                               
      |                                                                     
      | Place copyright information at the top of every subsystem in design.
      mask prompts: none "No parameters"
      mask help: Place copyright information at the top of every subsystem in design.
      mask Display:
      | NxtrConf = 'Nexteer Confidential';
      | 
      | sys = bdroot; %handle for the current model ("system")
      | first = get_param(sys,'Created');
      | first = first(end-3:end);  %year is last four digits
      | 
      | last = get_param(sys,'LastModifiedDate');
      | if isempty(last)
      |     last = datestr(now,'yyyy');
      | else
      |     last = last(end-3:end);
      | end
      | 
      | if strcmp(first,last)
      |     fprintf('%s -- Copyright %s Nexteer',NxtrConf,first)
      | else
      |     fprintf('%s -- %s%s- %s Nexteer',NxtrConf,char(169),first,last)
      | end
  Data Store Read : DataStoreRead  DataStoreName=RampYes
  Data Store Read1 : DataStoreRead  DataStoreName=RampNo
  Data Store Write1 : DataStoreWrite  DataStoreName=dWhlImbRejctnScaRi
  Data Store Write4 : DataStoreWrite  DataStoreName=dWhlImbRejctnScaLe
  Enable Ramp : Subsystem
  ScaleL : Outport
  ScaleR : Outport  Port=2
  Enable : Outport  Port=3
  WhlImbRejctnActv : Outport  Port=4
  wires:
  FreqEstAvg_Hz1/1 -> Calculate Enable1/1(FreqEstAvg_Hz)
  WhlSpdLFilt/1 -> Calculate Enable1/2(WhlSpdLFilt)
  WhlSpdRFilt/1 -> Calculate Enable1/3(WhlSpdRFilt)
  Calculate Enable1/2(ScaleR) -> Data Store Write1/1, ScaleR/1
  VehSpd/1 -> Calculate Enable1/4(Vehicle_Speed)
  VehspdValid/1 -> Calculate Enable1/5(Vehicle_Speed_Valid)
  WhlImbRejctnCustEna/1 -> Calculate Enable1/6(WhlImbRejctnCustEna)
  WhlImbRejctnDi/1 -> Calculate Enable1/7(WhlImbRejctnDi)
  Calculate Enable1/3(Enable) -> Enable Ramp/1(Enable In)
  Enable Ramp/1(Ramped Enable) -> Enable/1
  Calculate Enable1/1(ScaleL) -> Data Store Write4/1, ScaleL/1
  System_State/1 -> Enable Ramp/4(SYSTEM_STATE)
  Data Store Read/1 -> Enable Ramp/2("RampY ")
  Data Store Read1/1 -> Enable Ramp/3(RampN)
  Calculate Enable1/4(WhlImbRejctnActv) -> WhlImbRejctnActv/1
  CurrMgnSlewRate/1 -> Calculate Enable1/8(CurrMgnSlewRate)
  EnaSlewRate/1 -> Calculate Enable1/9(EnaSlewRate)
